simulink model "LQR_NL"  (R2019b)
settings: Solver=VariableStepAuto  StartTime=0.0  StopTime=1000  RelTol=1e-3
undefined symbols (not defined in the file): K
settings Model: Creator=Envy  LastModifiedBy=shubh
settings DataIOCC: ReturnWorkspaceOutputs=off
settings DebuggingCC: ArithmeticOperatorsInVariantConditions=warning
settings SFSimCC: CustomCodeUndefinedFunction=UseInterfaceOnly

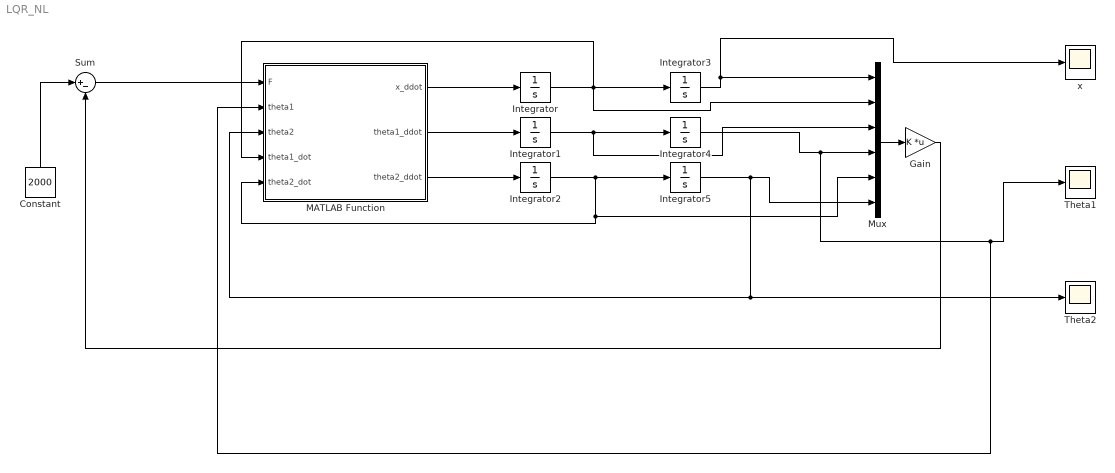
== system LQR_NL ==
  Constant : Constant  Value=2000
  Gain : Gain  Gain=K  Multiplication=Matrix(K*u)
  Integrator{,1..5} (6 alike) : Integrator
  MATLAB Function : MATLAB Function  TreatAsAtomicUnit=on
  Mux : Mux  Inputs=6
  Sum : Sum  Inputs=|+-
  Theta1 : Scope
  Theta2 : Scope
  x : Scope
  wires:
  Mux/1 -> Gain/1
  Sum/1 -> MATLAB Function/1(F)
  Constant/1 -> Sum/1
  Gain/1 -> Sum/2
  MATLAB Function/1(x_ddot) -> Integrator/1
  MATLAB Function/2(theta1_ddot) -> Integrator1/1
  MATLAB Function/3(theta2_ddot) -> Integrator2/1
  Integrator/1 -> Mux/2, MATLAB Function/4(theta1_dot), Integrator3/1
  Integrator1/1 -> Mux/3, Integrator4/1
  Integrator2/1 -> MATLAB Function/5(theta2_dot), Mux/5, Integrator5/1
  Integrator3/1 -> Mux/1, x/1
  Integrator5/1 -> MATLAB Function/3(theta2), Theta2/1, Mux/6
  Integrator4/1 -> MATLAB Function/2(theta1), Theta1/1, Mux/4

== matlab function LQR_NL/MATLAB Function ==
  data: F input; theta1 input; theta2 input; x_ddot output; theta1_dot input; theta2_dot input; theta1_ddot output; theta2_ddot output
function [x_ddot,theta1_ddot,theta2_ddot] = NL_SS(F,theta1,theta2,theta1_dot,theta2_dot)

M = 1000; 
m1 = 100; 
m2 = 100; 
l1 = 20; 
l2 = 10; 
g = 9.81;
%% x_ddot equation 
x_ddot = (F - m1*g*sin(theta1)*cos(theta1) - m2*g*sin(theta2)*cos(theta2) -m1*l1*(theta1_dot^2)*(sin(theta1)) - m2*l2*(theta2_dot^2)*(sin(theta2)))/(m1*(sin(theta1)^2) + m2*(sin(theta2)^2) + M);

%% Theta1_ddot equation
theta1_ddot = (x_ddot*cos(theta1) - g*sin(theta1))/l1;

%% Theta2_ddot equation
theta2_ddot = (x_ddot*cos(theta2) - g*sin(theta2))/l2;

end
